simulink model "p5p5c_model"  (Simulink 8.9)
settings: Solver=ode45  StartTime=0.0  StopTime=500  RelTol=1e-3  EnableMultiTasking=on
values from neighbouring files (symbols this model uses):
  Kpd = 0.8370    (= 0.837)    [p5p5c.m]    (also in p5p5d.m; p5p5e.m; p5p5e_fix.m)
  Td = T    (= 72.4637)    [p5p5c.m]    (also in p5p5d.m; p5p5e.m; p5p5e_fix.m)
  Tf = 8.402    [p5p5c.m]    (also in p5p5d.m; p5p5e.m; p5p5e_fix.m)
  Ts = 0.1    [p5p5c.m]    (also in p5p5d.m; p5p5e.m; p5p5e_fix.m)
libraries: simulink_extras x7, simulink x2
settings Model: Creator=markh  LastModifiedBy=sondrna
settings DataIOCC: SignalLoggingName=sigsOut
settings OptimizationCC: InitFltsAndDblsToZero=on
settings DebuggingCC: SaveWithParameterizedLinksMsg=none  SignalResolutionControl=TryResolveAllWithWarning  MultiTaskDSMMsg=warning  MultiTaskCondExecSysMsg=none
settings HardwareCC: TargetUnknown=on
settings GRTTargetCC: TargetFcnLib=ansi_tfl_tmw.mat

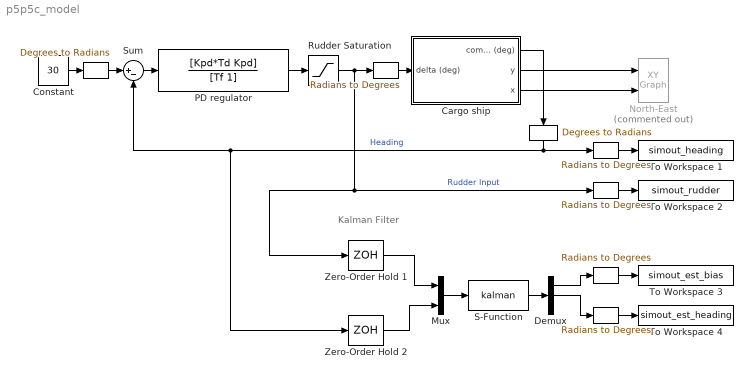
== system p5p5c_model ==
  note: Kalman Filter
  " " : simulink_extras/Transformations/Degrees to Radians
  "  " : simulink_extras/Transformations/Degrees to Radians
  "   " : simulink_extras/Transformations/Radians to Degrees
  "    " : simulink_extras/Transformations/Radians to Degrees
  "     " : simulink_extras/Transformations/Radians to Degrees
  "      " : simulink_extras/Transformations/Radians to Degrees
  "       " : simulink_extras/Transformations/Radians to Degrees
  Cargo ship : Subsystem  mask(Simple shipmodel for a cargo ship){noise=on, current=on, logic=on}
      mask prompts: noise "measurement noise"; logic "waves"
      mask help:
      | Measurement noise:
      | 	checked = noise on
      | 	unchecked = noise off
      |
      | Current:
      | 	checked = current on
      | 	unchecked = current off
      |
      | Waves:
      | 	checked = waves on
      | 	unchecked = waves off
      |
      | Author: Jørgen Spjøtvold, 9/10-2003
      | TTK 4115 Linear system theory.
      | Modified by Jostein Bakkeheim 26/10-2006
  Constant : Constant  Value=30
  Demux : Demux  Outputs=3
  Mux : Mux  Inputs=2
  North-East : simulink/Sinks/XY Graph  Commented=on  xmin=-5000  xmax=5000  ymin=-5000  ymax=5000  st=-1
  PD regulator : TransferFcn  Numerator=[Kpd*Td Kpd]  Denominator=[Tf 1]
  Rudder Saturation : Saturate  UpperLimit=45*(pi/180)  LowerLimit=-45*(pi/180)
  S-Function : S-Function  FunctionName=kalman  Parameters=data  SFunctionDeploymentMode=off  EnableBusSupport=off
  Sum : Sum  Inputs=|+-
  To Workspace 1 : ToWorkspace  VariableName=simout_heading  SaveFormat=Timeseries  SampleTime=-1
  To Workspace 2 : ToWorkspace  VariableName=simout_rudder  SaveFormat=Timeseries  SampleTime=-1
  To Workspace 3 : ToWorkspace  VariableName=simout_est_bias  SaveFormat=Timeseries  SampleTime=-1
  To Workspace 4 : ToWorkspace  VariableName=simout_est_heading  SaveFormat=Timeseries  SampleTime=-1
  Zero-Order Hold 1 : ZeroOrderHold  SampleTime=Ts
  Zero-Order Hold 2 : ZeroOrderHold  SampleTime=Ts
  wires:
  Cargo ship/3(x) -> North-East/2
  Cargo ship/2(y) -> North-East/1
  Sum/1 -> PD regulator/1
  "   "/1 -> Cargo ship/1(delta (deg))
  Rudder Saturation/1 -> "     "/1, Zero-Order Hold 1/1, "   "/1  "Rudder Input"
  Constant/1 -> " "/1
  PD regulator/1 -> Rudder Saturation/1
  "  "/1 -> Zero-Order Hold 2/1, Sum/2, "    "/1  "Heading"
  Cargo ship/1(compass (deg)) -> "  "/1
  " "/1 -> Sum/1
  Demux/2 -> "       "/1
  Demux/1 -> "      "/1
  Zero-Order Hold 2/1 -> Mux/2
  Zero-Order Hold 1/1 -> Mux/1
  S-Function/1 -> Demux/1
  Mux/1 -> S-Function/1
  "    "/1 -> To Workspace 1/1
  "     "/1 -> To Workspace 2/1
  "      "/1 -> To Workspace 3/1
  "       "/1 -> To Workspace 4/1

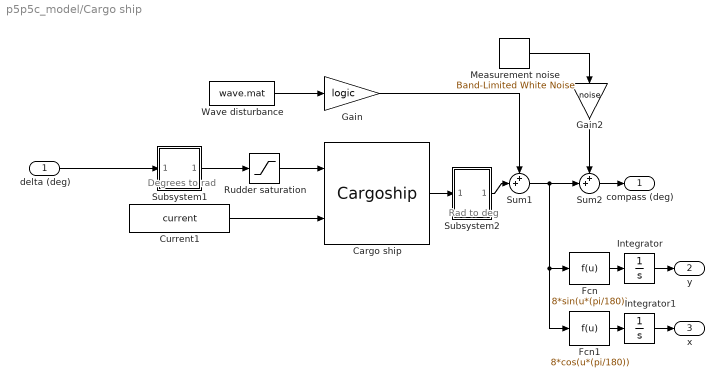
== system p5p5c_model/Cargo ship ==
  note: Degrees to rad
  note: Rad to deg
  delta (deg) : Inport
  Cargo ship : S-Function  FunctionName=Cargoship  SFunctionDeploymentMode=off  EnableBusSupport=off  mask(Cargo ship){}
      mask help:
      | S-function which simulates a cargo ship.
      |
      | Author: Jørgen Spjøtvold
      | 20.10-2003
      | Modified by Jostein Bakkeheim 27.10.2006
  Current1 : Constant  Value=current
  Fcn : Fcn  Expr=8*sin(u*(pi/180))
  Fcn1 : Fcn  Expr=8*cos(u*(pi/180))
  Gain : Gain  Gain=logic  SaturateOnIntegerOverflow=on  OutDataTypeStr=Inherit: Same as input  ParamDataTypeStr=Inherit: Same as input
  Gain2 : Gain  Gain=noise  SaturateOnIntegerOverflow=on  OutDataTypeStr=Inherit: Same as input  ParamDataTypeStr=Inherit: Same as input
  Integrator : Integrator
  Integrator1 : Integrator
  Measurement noise : simulink/Sources/Band-Limited White Noise  Cov=[0.001]  Ts=.5  seed=[23341]
  Rudder saturation : Saturate  UpperLimit=45*(pi/180)  LowerLimit=-45*(pi/180)
  Subsystem1 : Subsystem  mask(degrees to radians){}
      mask help: Converts degrees to radians
      mask Display: fprintf('D2R');
  Subsystem2 : Subsystem  mask(radians to degrees){}
      mask help: Converts radians to degrees
      mask Display: fprintf('R2D');
  Sum1 : Sum  Inputs=++|  SaturateOnIntegerOverflow=on
  Sum2 : Sum  Inputs=++|  SaturateOnIntegerOverflow=on
  Wave disturbance : FromFile  FileName=wave.mat  SampleTime=0
  compass (deg) : Outport
  y : Outport  Port=2
  x : Outport  Port=3
  wires:
  delta (deg)/1 -> Subsystem1/1(In1)
  Fcn/1 -> Integrator/1
  Integrator/1 -> y/1
  Fcn1/1 -> Integrator1/1
  Integrator1/1 -> x/1
  Wave disturbance/1 -> Gain/1
  Subsystem2/1(Out1) -> Sum1/2
  Gain/1 -> Sum1/1
  Sum1/1 -> Fcn/1, Fcn1/1, Sum2/2
  Cargo ship/1 -> Subsystem2/1(In1)
  Subsystem1/1(Out1) -> Rudder saturation/1
  Rudder saturation/1 -> Cargo ship/1
  Sum2/1 -> compass (deg)/1
  Measurement noise/1 -> Gain2/1
  Gain2/1 -> Sum2/1
  Current1/1 -> Cargo ship/2

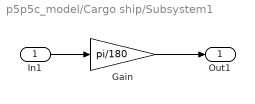
== system p5p5c_model/Cargo ship/Subsystem1 ==
  In1 : Inport
  Gain : Gain  Gain=pi/180  SaturateOnIntegerOverflow=on  OutDataTypeStr=Inherit: Same as input  ParamDataTypeStr=Inherit: Same as input
  Out1 : Outport
  wires:
  Gain/1 -> Out1/1
  In1/1 -> Gain/1

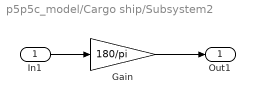
== system p5p5c_model/Cargo ship/Subsystem2 ==
  In1 : Inport
  Gain : Gain  Gain=180/pi  SaturateOnIntegerOverflow=on  OutDataTypeStr=Inherit: Same as input  ParamDataTypeStr=Inherit: Same as input
  Out1 : Outport
  wires:
  Gain/1 -> Out1/1
  In1/1 -> Gain/1
